simulink model "Ex2"  (R2021b)
settings: Solver=FixedStepAuto  StartTime=0.0  StopTime=0.2e-6  FixedStep=1e-9  RelTol=1e-3
values from neighbouring files (symbols this model uses):
  AT = [-R/L -1/L;1/C 0]    [Ex2_comp.m]
  BT = [1/L;0]    [Ex2_comp.m]
  CT = [1 0;0 1]    [Ex2_comp.m]
  DT = 0    [Ex2_comp.m]
settings Model: Creator=gaeta  LastModifiedBy=gaeta

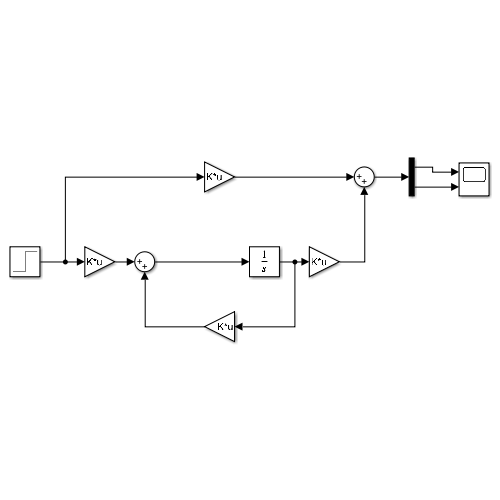
[thumbnail: Simulink's stored preview of the top-level diagram]
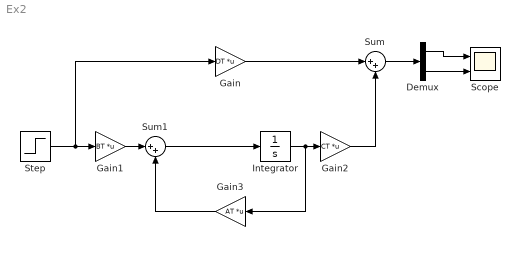
== system Ex2 ==
  Demux : Demux  Outputs=2
  Gain : Gain  Gain=DT  Multiplication=Matrix(K*u)
  Gain1 : Gain  Gain=BT  Multiplication=Matrix(K*u)
  Gain2 : Gain  Gain=CT  Multiplication=Matrix(K*u)
  Gain3 : Gain  Gain=AT  Multiplication=Matrix(K*u)
  Integrator : Integrator
  Scope : Scope  NumInputPorts=2
  Step : Step  Time=1e-8  After=1e-6  SampleTime=0
  Sum : Sum  Inputs=|++
  Sum1 : Sum  Inputs=|++
  wires:
  Gain/1 -> Sum/1
  Step/1 -> Gain1/1, Gain/1
  Sum1/1 -> Integrator/1
  Gain1/1 -> Sum1/1
  Gain2/1 -> Sum/2
  Gain3/1 -> Sum1/2
  Integrator/1 -> Gain3/1, Gain2/1
  Sum/1 -> Demux/1
  Demux/1 -> Scope/1
  Demux/2 -> Scope/2
